simulink model "RollControlSimulationV2"  (R2021a)
settings: Solver=VariableStepAuto  StartTime=0.0  StopTime=10.0  RelTol=1e-3
values from neighbouring files (symbols this model uses):
  C = derivada_coef_D_aletas + derivada_coef_D_canards    (= 37.955768493)    [RollControlParameters.m]
  J = 0.030    (= 0.03)    [RollControlParameters.m]
  Kdelta = DynamicPressure*Ar*Lr*(derivada_coef_f_aletas-derivada_coef_f_canards)    (= 85.6979576796)    [RollControlParameters.m]
  P = DynamicPressure * Ar * Lr * Lr / 2 / speed    (= 0.00357793574932)    [RollControlParameters.m]
libraries: slpidlib x1
settings Model: Creator=wujia  LastModifiedBy=wujia

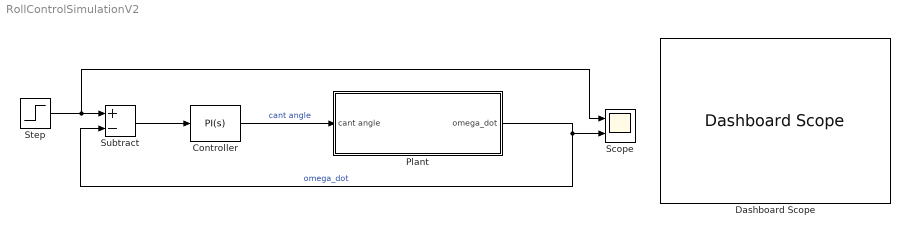
== system RollControlSimulationV2 ==
  Controller : slpidlib/PID Controller  Controller=PI  Form=Parallel  TimeDomain=Continuous-time  UseExternalTs=off  SampleTime=-1  IntegratorMethod=Forward Euler  FilterMethod=Forward Euler  ControllerParametersSource=internal  P=0.17  I=0.0315  D=0  UseFilter=on  N=100  TunerSelectOption=Transfer Function Based (PID Tuner App)  InitialConditionSource=internal  InitialConditionForIntegrator=0  InitialConditionForFilter=0  DifferentiatorICPrevScaledInput=0  ExternalReset=none  TrackingMode=off  Kt=1  LimitOutput=on  SatLimitsSource=internal  UpperSaturationLimit=8  LowerSaturationLimit=-8  LinearizeAsGain=on  AntiWindupMode=clamping  Kb=1  POutMin=[]  POutMax=[]  IOutMin=[]  IOutMax=[]  DOutMin=[]  DOutMax=[]  NOutMin=[]  NOutMax=[]  SumOutMin=[]  SumOutMax=[]  SaturationOutMin=[]  SaturationOutMax=[]  PParamMin=[]  PParamMax=[]  IParamMin=[]  IParamMax=[]  DParamMin=[]  DParamMax=[]  NParamMin=[]  NParamMax=[]  KbParamMin=[]  KbParamMax=[]  KtParamMin=[]  KtParamMax=[]  KbOutMin=[]  KbOutMax=[]  KtOutMin=[]  KtOutMax=[]  IntegratorOutMin=[]  IntegratorOutMax=[]  FilterOutMin=[]  FilterOutMax=[]  SumI1OutMin=[]  SumI1OutMax=[]  SumI2OutMin=[]  SumI2OutMax=[]  SumI3OutMin=[]  SumI3OutMax=[]  SumI4OutMin=[]  SumI4OutMax=[]  SumDOutMin=[]  SumDOutMax=[]  DifferentiatorOutMin=[]  DifferentiatorOutMax=[]  FilterDiffOutCoefMin=[]  FilterDiffOutCoefMax=[]  ReciprocalOutMin=[]  ReciprocalOutMax=[]  SumDenOutMin=[]  SumDenOutMax=[]  SumNumOutMin=[]  SumNumOutMax=[]  DivideOutMin=[]  DivideOutMax=[]  UdiffTsProdOutMin=[]  UdiffTsProdOutMax=[]  NTsProdOutMin=[]  NTsProdOutMax=[]  UintegralTsProdOutMin=[]  UintegralTsProdOutMax=[]  UngainTsProdOutMin=[]  UngainTsProdOutMax=[]  IntegratorContinuousStateAttributes=''  IntegratorStateMustResolveToSignalObject=off  IntegratorRTWStateStorageClass=Auto  FilterContinuousStateAttributes=''  FilterStateMustResolveToSignalObject=off  FilterRTWStateStorageClass=Auto  ParallelPVariant=InternalParameters  IdealPVariant=Disabled  IVariant=InternalParameters  DVariant=Disabled  IntegratorVariant=Continuous  SatVariant=Enabled  AWVariant=ContClampingParallel  PCopyVariant=Disabled  TRVariant=Disabled  FdbkBlocksVariant=Forward  IdealPFdbkVariant=Disabled  SatFdbkVariant=Disabled  DerivativeFilterVariant=Disabled  NVariant=Disabled  NCopyVariant=Disabled_SignalSpec  FilterICVariant=Disabled  IntegratorICVariant=InternalICs  ExternalResetVariant=Disabled  TRSumVariant=Passthrough  SumFdbkVariant=Disabled  SumVariant=Sum_PI  TsampFilterVariant=InternalTs  TsampNgainVariant=Passthrough  TsampIntegralVariant=Passthrough  ExternalSaturationOutDataTypeStr=Inherit: Same as second input
  Dashboard Scope : DashboardScope
  Plant : Subsystem
  Scope : Scope  NumInputPorts=2
  Step : Step  SampleTime=0
  Subtract : Sum  Inputs=+-
  wires:
  Controller/1 -> Plant/1(cant angle)  "cant angle"
  Plant/1(omega_dot) -> Subtract/2, Scope/2  "omega_dot"
  Subtract/1 -> Controller/1
  Step/1 -> Scope/1, Subtract/1

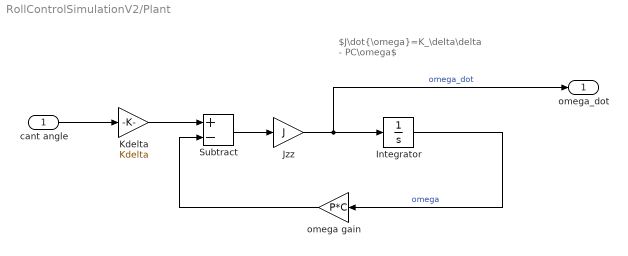
== system RollControlSimulationV2/Plant ==
  note: $J\dot{\omega}=K_\delta\delta - PC\omega$
  cant angle : Inport
  Integrator : Integrator
  Jzz : Gain  Gain=J
  Kdelta : Gain  Gain=Kdelta
  Subtract : Sum  Inputs=+-
  omega gain : Gain  Gain=P*C
  omega_dot : Outport
  wires:
  Jzz/1 -> omega_dot/1, Integrator/1  "omega_dot"
  Kdelta/1 -> Subtract/1
  omega gain/1 -> Subtract/2
  cant angle/1 -> Kdelta/1
  Subtract/1 -> Jzz/1
  Integrator/1 -> omega gain/1  "omega"
